simulink library "GOcontroll_Moduline_Target"  (R2023b)
settings: Solver=ode45  StartTime=0.0  StopTime=10.0  RelTol=1e-3  EnableMultiTasking=on
PreLoadFcn:
  | compile_gocontroll_mex;
values from neighbouring files (symbols this model uses):
  id = 2    [sfcn_UDPReceive.m]    (also in sfcn_UDPSend.m = 4)
undefined symbols (not defined in the file or in its folder): C_Cb1Pt10, Cb1Pt10_RAW_ERR_HIGH, Cb1Pt10_RAW_ERR_LOW, Cb1Pt10_SIG_ERR_HIGH, Cb1Pt10_SIG_ERR_LOW, Cb1Pt10_SIG_WAR_HIGH, Cb1Pt10_SIG_WAR_LOW, Pres_0_20_bar_500_4500_mv_inv, signal_x_RAW_ERR_HIGH, signal_x_RAW_ERR_LOW, signal_x_SIG_ERR_HIGH, signal_x_SIG_ERR_LOW, signal_x_SIG_WAR_HIGH, signal_x_SIG_WAR_LOW, signal_x_SPN, Valve1_ACTIVE_DUTY_CYCLE, Valve1_MAX_CURRENT, Valve1_MIN_CURRENT, Valve1_SPN
libraries: $bdroot x17, simulink x12, canmsglib x4
(part 4 of 5)

== system GOcontroll_Moduline_Target/Network/TCP ==
  TCP Configure : M-S-Function  FunctionName=sfcn_TCPConfig  mask(TCP Configure){socket_id=id, port=9001, ip='0.0.0.0', socket_mode=Server, remote_port=9002, remote_ip='0.0.0.0', timeout=1000}
      mask prompts: socket_id "Socket id"; port "The port on which to listen/send"; ip "The ip on which to listen/send"; socket_mode "Socket mode:"; remote_port "The port to connect to"; remote_ip "The ip to connect to"; timeout "The connection timeout (ms)"
      mask help:
      | Block to configure a TCP socket
      |
      | The socket ID should be a unique identifier to link the send and receive blocks to.
      | The name of the actual socket in the C code will be socket_<socket id>, so characters that would not work in a C variable name will not work.
      |
      | Setting the ip to 0.0.0.0 makes the controller accept messages on all interfaces.
      | Set it to the ip of a specific interface to limit this.
      |
      | The socket mode determines whether this socket will listen for a connection or actively try to make one to a given ip and port.
      | Server will wait for something to connect to it, the client will try to connect to a server at the given ip and port
      |
      | Setting the timeout to zero disables the timeout
      |
      | When the disconnect input is true, it will close the current connection if there is one, if there isn't one it will not allow a connection to be made as long as it is true.
      |
      | Outputs whether or not the socket currently has an active connection (true means connnected)
      mask init:
      | if ~is_ip(ip)
      |         error('Entered IP is not valid');
      |     end
      |     if mod(port,1) > 0 || port < intmin('uint16') || port > intmax('uint16')
      |         error('Entered Port is not valid, it should be an integer from 0-65335');
      |     end
      | 
      |     if ~is_ip(remote_ip)
      |         error('Entered remote IP is not valid');
      |     end
      |     if mod(remote_port,1) > 0 || remote_port < intmin('uint16') || remote_port > intmax('uint16')
      |         error('Entered remote Port is not valid, it should be an integer from 0-65335');
      |     end
      | 
      |     if mod(timeout,1) > 0 || timeout < intmin('uint32') || timeout > intmax('uint32')
      |         error('Entered timeout is not valid, it should be an integer from 0-4.294.967.295');
      |     end
      | 
      |     blockPath = split(gcb, '/');
      |     configures = find_system(blockPath(1),'RegExp', 'on','FollowLinks', 'on','MaskType','TCP Configure');
      |     options = cell(1,length(configures));
      |     for idx = 1:length(configures)
      |         options(idx) = get_param(configures(idx),'socket_id');
      |     end
      | 
      |     if length(unique(options)) ~= length(options)
      |         error('Socket id is already in use, set a unique socket id');
      |     end
      | 
      | 	modelRTWFields = struct('port', num2str(port), 'ip', ip, 'socket_id', socket_id, ...
      |         'remote_port', num2str(remote_port), 'remote_ip', remote_ip, 'socket_mode', num2str(socket_mode), 'timeout', num2str(timeout));
      | 
      | 	% Insert modelRTWFields in the I/O block S-Function containing the Tag starting with 'HANcoder_TARGET_'
      | 	HANcoder_TARGET_DataBlock = find_system(gcb, 'RegExp', 'on', 'FollowLinks', 'on', 'LookUnderMasks', 'all', 'BlockType', 'M-S-Function');
      | 	set_param(HANcoder_TARGET_DataBlock{1}, 'RTWdata', modelRTWFields);
      mask TypeOptions socket_mode: Server | Client
      mask Callback socket_mode:
      | mode = get_param(gcb, 'socket_mode');
      | mask = Simulink.Mask.get(gcb);
      | pars = mask.Parameters;
      | if strcmp(mode, 'Server')
      |     pars(5).set('Visible', 'off');
      |     pars(6).set('Visible', 'off');
      | else
      |     pars(5).set('Visible', 'on');
      |     pars(6).set('Visible', 'on');
      | end
      mask Display:
      | if (socket_mode == 1)
      |     fprintf('Configure TCP server\n IP: %s\nPort: %d',ip,port);
      | else
      |     fprintf('Configure TCP client\n IP: %s\nPort: %d\nRemote IP: %s\n Remote port: %d',ip,port,remote_ip,remote_port);
      | end
      | port_label('output', 1, 'connected');
      | port_label('input', 1, 'disconnect');
      | text(2, 6, ert_linux_target_version());
  TCP Receive : S-Function  FunctionName=sfcn_TCPReceive  Parameters=buff_len,socket_mode,socket_id,tsamp  SFunctionDeploymentMode=off  EnableBusSupport=off  mask(TCP Receive){tsamp=-1, socket_id=id, buff_len=1, socket_mode=Server}
      mask prompts: tsamp "Sample time"; socket_id "Socket"; buff_len "Buffer size"
      mask help:
      | Receive all TCP messages on the given socket
      |
      | For every message received this block will call the functions attached to the function call output.
      | In these function calls you can then use the message and message length outputs to process/buffer the received messages.
      |
      | Outputs:
      | function call:
      | Attach to a function call subsystem or something like it to call that function every time a message is received.
      |
      | message:
      | The uint8 vector received from the socket. The length of this vector is likely longer than the actual number of bytes received.
      |
      | message length:
      | The number of bytes actually received, use this to get the actual fresh bytes from the message.
      |
      | Parameters:
      | buffer size:
      | The maximum number of bytes that can be read from the socket in one message, this also determines the width of the message vector.
      mask TypeOptions socket_id: id
      mask Callback socket_id:
      | blockPath = split(gcb, '/');
      | configures = find_system(blockPath(1),'RegExp', 'on','FollowLinks', 'on','MaskType','TCP Configure');
      | mask = Simulink.Mask.get(gcb);
      | pars = mask.Parameters;
      | options = cell(1,length(configures));
      | for idx = 1:length(configures)
      |     options(idx) = get_param(configures(idx),'socket_id');
      | end
      | mask.getParameter('socket_id').TypeOptions = options;
      | for idx = 1:length(configures)
      |     if strcmp(get_param(configures(idx),'socket_id'), get_param(gcb, 'socket_id'))
      |         mode = Simulink.Mask.get(configures{idx}).getParameter('socket_mode').Value;
      |         set_param(gcb, 'socket_mode', mode);
      |     end
      | end
      mask TypeOptions socket_mode: Server | Client
      mask Display:
      | fprintf('TCP Receive\nSocket: %s', socket_id);
      | text(2, 6, ert_linux_target_version());
      | port_label('output', 1, 'function call');
      | port_label('output', 2, 'message');
      | port_label('output', 3, 'message length');
  TCP Send : M-S-Function  FunctionName=sfcn_TCPSend  Parameters=tsamp  mask(TCP Send){socket_id=id, tsamp=1, socket_mode=Server}
      mask prompts: socket_id "Socket"; tsamp "Sample time"
      mask help:
      | Send a TCP message to the chosen sockets connection, whether it be client or server.
      |
      | The Message input should be a uint8 vector, if you end up with a [1xn] or [nx1] matrix, use the reshape block to turn it into a vector.
      mask init:
      | % update RTWdata to call WriteRTW again
      |     modelRTWFields = struct('socket_id', socket_id, 'socket_mode', num2str(socket_mode));
      | 
      |     % Insert modelRTWFields in the I/O block S-Function containing the Tag starting with 'HANcoder_TARGET_'
      |     HANcoder_TARGET_DataBlock = find_system(gcb, 'RegExp', 'on', 'FollowLinks', 'on', 'LookUnderMasks', 'all', 'BlockType', 'M-S-Function');
      |     set_param(HANcoder_TARGET_DataBlock{1}, 'RTWdata', modelRTWFields);
      mask TypeOptions socket_id: id
      mask Callback socket_id:
      | blockPath = split(gcb, '/');
      | configures = find_system(blockPath(1),'RegExp', 'on','FollowLinks', 'on','MaskType','TCP Configure');
      | mask = Simulink.Mask.get(gcb);
      | pars = mask.Parameters;
      | options = cell(1,length(configures));
      | for idx = 1:length(configures)
      |     options(idx) = get_param(configures(idx),'socket_id');
      | end
      | mask.getParameter('socket_id').TypeOptions = options;
      | for idx = 1:length(configures)
      |     if strcmp(get_param(configures(idx),'socket_id'), get_param(gcb, 'socket_id'))
      |         mode = Simulink.Mask.get(configures{idx}).getParameter('socket_mode').Value;
      |         set_param(gcb, 'socket_mode', mode);
      |     end
      | end
      mask TypeOptions socket_mode: Server | Client
      mask Display:
      | fprintf('TCP Send\nSocket: %s',socket_id);
      | port_label('input', 1, 'message');
      | text(2, 6, ert_linux_target_version());

== system GOcontroll_Moduline_Target/Network/UDP ==
  UDP Configure : M-S-Function  FunctionName=sfcn_UDPConfig  mask(UDP Configure){socket_id=id, port=9001, ip='0.0.0.0', broadcast=on}
      mask prompts: socket_id "Socket id"; port "The port on which to listen/send"; ip "The ip on which to listen/send"; broadcast "Allow broadcasting of sent messages"
      mask help:
      | Block to configure a UDP connection
      |
      | The socket ID should be a unique identifier to link the send and receive blocks to.
      | The name of the actual socket in the C code will be socket_<socket id>, so characters that would not work in a C variable name will not work.
      |
      | Setting the ip to 0.0.0.0 makes the controller accept messages on all interfaces.
      | Set it to the ip of a specific interface to limit this.
      |
      | Allowing broadcasting enables you to send messages to a full range of ip addresses, for example:
      | 192.168.255.255 sends messages to 192.168.1.1, 192.168.2.1 ... 192.168.1.2, 192.168.1.3...
      mask init:
      | if broadcast == 0
      |         broadcastStr = "Not broadcasting";
      |     else
      |         broadcastStr = "Broadcasting";
      |     end
      |     if ~is_ip(ip)
      |         error('Entered IP is not valid');
      |     end
      |     if mod(port,1) > 0 || port < intmin('uint16') || port > intmax('uint16')
      |         error('Entered Port is not valid, it should be an integer from 0-65335');
      |     end
      | 
      |     blockPath = split(gcb, '/');
      |     configures = find_system(blockPath(1),'RegExp', 'on','FollowLinks', 'on','MaskType','UDP Configure');
      |     options = cell(1,length(configures));
      |     for idx = 1:length(configures)
      |         options(idx) = get_param(configures(idx),'socket_id');
      |     end
      | 
      |     if length(unique(options)) ~= length(options)
      |         error('Socket id is already in use, set a unique socket id');
      |     end
      | 
      | 	modelRTWFields = struct('port', num2str(port), 'ip', ip, 'broadcast', num2str(broadcast), 'socket_id', socket_id);
      | 
      | 	% Insert modelRTWFields in the I/O block S-Function containing the Tag starting with 'HANcoder_TARGET_'
      | 	HANcoder_TARGET_DataBlock = find_system(gcb, 'RegExp', 'on', 'FollowLinks', 'on', 'LookUnderMasks', 'all', 'BlockType', 'M-S-Function');
      | 	set_param(HANcoder_TARGET_DataBlock{1}, 'RTWdata', modelRTWFields);
      mask Display:
      | fprintf('Configure UDP socket\n IP: %s\nPort: %d\n%s',ip,port,broadcastStr);
      | text(2, 6, ert_linux_target_version());
  UDP Example : Subsystem
  UDP Receive : S-Function  FunctionName=sfcn_UDPReceive  Parameters=buff_len,socket_id,tsamp  SFunctionDeploymentMode=off  EnableBusSupport=off  mask(UDP Receive){tsamp=-1, socket_id=id, buff_len=1}
      mask prompts: tsamp "Sample time"; socket_id "Socket"; buff_len "Buffer size"
      mask help:
      | Receive all UDP messages
      |
      | For every message received this block will call the functions attached to the function call output.
      | In these function calls you can then use the message and message length outputs to process/buffer the received messages.
      |
      | Outputs:
      | function call:
      | Attach to a function call subsystem or something like it to call that function every time a message is received.
      |
      | message:
      | The uint8 vector received from the socket. The length of this vector is likely longer than the actual number of bytes received.
      |
      | message length:
      | The number of bytes actually received, use this to get the actual fresh bytes from the message.
      |
      | Parameters:
      | buffer size:
      | The maximum number of bytes that can be read from the socket in one message, this also determines the width of the message vector.
      mask TypeOptions socket_id: id | led_sinus
      mask Callback socket_id:
      | blockPath = split(gcb, '/');
      | configures = find_system(blockPath(1),'RegExp', 'on','FollowLinks', 'on','MaskType','UDP Configure');
      | mask = Simulink.Mask.get(gcb);
      | pars = mask.Parameters;
      | options = cell(1,length(configures));
      | for idx = 1:length(configures)
      |     options(idx) = get_param(configures(idx),'socket_id');
      | end
      | mask.getParameter('socket_id').TypeOptions = options;
      mask Display:
      | fprintf('UDP Receive');
      | text(2, 6, ert_linux_target_version());
      | port_label('output', 1, 'function call');
      | port_label('output', 2, 'message');
      | port_label('output', 3, 'message length');
  UDP Send : M-S-Function  FunctionName=sfcn_UDPSend  Parameters=tsamp,ip,port  mask(UDP Send){socket_id=id, ip='0.0.0.0', port=9001, tsamp=1}
      mask prompts: socket_id "Socket"; ip "The IP address to send to"; port "The port to send to"; tsamp "Sample time"
      mask help:
      | Send a UDP message to the designated address.
      |
      | The Message input should be a uint8 vector, if you end up with a [1xn] or [nx1] matrix, use the reshape block to turn it into a vector.
      |
      | IP address should be a valid IP address as a string
      |
      | Port should be a within the range of a uint16
      mask init:
      | if ~is_ip(ip)
      |         error('Entered IP is not valid');
      |     end
      |     if mod(port,1) > 0 || port < intmin('uint16') || port > intmax('uint16')
      |         error('Entered Port is not valid, it should be an integer from 0-65335');
      |     end
      |     % update RTWdata to call WriteRTW again
      |     modelRTWFields = struct('port', num2str(port), 'ip', ip, 'socket_id', socket_id);
      | 
      |     % Insert modelRTWFields in the I/O block S-Function containing the Tag starting with 'HANcoder_TARGET_'
      |     HANcoder_TARGET_DataBlock = find_system(gcb, 'RegExp', 'on', 'FollowLinks', 'on', 'LookUnderMasks', 'all', 'BlockType', 'M-S-Function');
      |     set_param(HANcoder_TARGET_DataBlock{1}, 'RTWdata', modelRTWFields);
      mask TypeOptions socket_id: id | led_sinus
      mask Callback socket_id:
      | blockPath = split(gcb, '/');
      | configures = find_system(blockPath(1),'RegExp', 'on','FollowLinks', 'on','MaskType','UDP Configure');
      | mask = Simulink.Mask.get(gcb);
      | pars = mask.Parameters;
      | options = cell(1,length(configures));
      | for idx = 1:length(configures)
      |     options(idx) = get_param(configures(idx),'socket_id');
      | end
      | pars(1).TypeOptions = options;
      mask Display:
      | fprintf('UDP Send\nIP: %s\nPort: %d',ip,port);
      | port_label('input', 1, 'message');
      | text(2, 6, ert_linux_target_version());

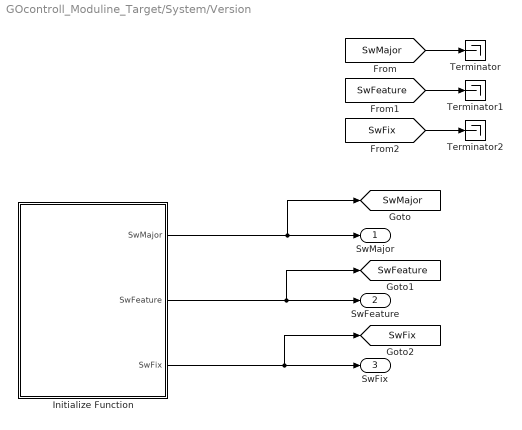
== system GOcontroll_Moduline_Target/System/Version ==
  Initialize Function : Subsystem  TreatAsAtomicUnit=on
  Terminator : Terminator
  Terminator1 : Terminator
  Terminator2 : Terminator
  SwMajor : Outport
  SwFeature : Outport  Port=2
  SwFix : Outport  Port=3
  tag scope: SwFeature=global, SwFix=global, SwMajor=global
  wires:
  Initialize Function/2(SwFeature) -> [SwFeature], SwFeature/1
  Initialize Function/1(SwMajor) -> SwMajor/1, [SwMajor]
  Initialize Function/3(SwFix) -> [SwFix], SwFix/1
  [SwMajor] -> Terminator/1
  [SwFeature] -> Terminator1/1
  [SwFix] -> Terminator2/1

== system GOcontroll_Moduline_Target/CAN/ CAN Example/Process messages on CAN2 ==
  note: only control the leds when a message has come in, so use enabled subystems
  note: place all your unpack blocks here attached to the CAN_MESSAGE line
  note: status outputs whether a message has been received the last time the block was activated
  In1 : Inport
  function : TriggerPort  TriggerType=function-call  VariantControl=(inherit)  OutputDataType=int8
  CAN Unpack : canmsglib/CAN Unpack  MsgList=(none)  MsgName=CAN Msg  MsgIDType=Standard (11-bit identifier)  MsgIdentifier=10  MsgLength=2  SignalInfo={ 'led1', '0', '8', 'LE', 'unsigned', 'Standard', '0', '1', '0', '-Inf', 'Inf'; 'led2', '8', '8', 'LE', 'unsigned', 'Standard', '0', '1', '0', '-Inf', 'Inf' }  IDPort=off  TimestampPort=off  ErrorPort=off  RemotePort=off  LengthPort=off  StatusPort=on  ApplyMinMax=off
      settings: LibrarySourceBlock=embeddedtargetslib/Host Communication/CAN Unpack
  CAN Unpack1 : canmsglib/CAN Unpack  MsgList=(none)  MsgName=CAN Msg  MsgIDType=Standard (11-bit identifier)  MsgIdentifier=11  MsgLength=2  SignalInfo={ 'led3', '0', '8', 'LE', 'unsigned', 'Standard', '0', '1', '0', '-Inf', 'Inf'; 'led4', '8', '8', 'LE', 'unsigned', 'Standard', '0', '1', '0', '-Inf', 'Inf' }  IDPort=off  TimestampPort=off  ErrorPort=off  RemotePort=off  LengthPort=off  StatusPort=on  ApplyMinMax=off
      settings: LibrarySourceBlock=embeddedtargetslib/Host Communication/CAN Unpack
  Control Leds : Subsystem  TreatAsAtomicUnit=on
  Enabled Subsystem : Subsystem  TreatAsAtomicUnit=on
  wires:
  CAN Unpack1/1 -> Enabled Subsystem/1(In4)
  CAN Unpack1/2 -> Enabled Subsystem/2(In2)
  CAN Unpack1/3 -> Enabled Subsystem/Enable
  CAN Unpack/3 -> Control Leds/Enable
  CAN Unpack/1 -> Control Leds/1(In1)
  CAN Unpack/2 -> Control Leds/2(In3)
  In1/1 -> CAN Unpack/1, CAN Unpack1/1

== system GOcontroll_Moduline_Target/Memory store/Diagnostic to memory/Delete all codes for one group ==
  Trigger : TriggerPort  VariantControl=(inherit)  PortDimensions=1
  Delete all DTC from memory : M-S-Function  FunctionName=sfcn_memory_diagnostic_delete_code  mask(Delete diagnostic codes from memory){}
      mask help:
      | This function block deletes all stored codes.
      |
      | Sample time:
      | -1 for inherited since this block is a triggered system
      mask init:
      | % Insert modelRTWFields in the I/O block S-Function containing the Tag starting with 'HANcoder_TARGET_'
      | HANcoder_TARGET_DataBlock = find_system(gcb, 'RegExp', 'on', 'FollowLinks', 'on', 'LookUnderMasks', 'all', 'BlockType', 'M-S-Function');
      mask Display:
      | fprintf('Delete all DTCs from memory');
      | text(2, 6, ert_linux_target_version());

== system GOcontroll_Moduline_Target/Memory store/Diagnostic to memory/Delete single DTC code ==
  In1 : Inport
  In2 : Inport  Port=2
  Trigger : TriggerPort  VariantControl=(inherit)
  Delete diagnostic code : M-S-Function  FunctionName=sfcn_memory_diagnostic_delete_single_code  mask(Store diagnostic code to memory){}
      mask help:
      | This function block stores a diagnostic code to memory.
      |
      | Diagnostic code type:
      | The type defines the severity of the diagnostic code.
      |
      | This block should be placed in a triggered subsystem
      mask init:
      | % Insert modelRTWFields in the I/O block S-Function containing the Tag starting with 'HANcoder_TARGET_'
      | HANcoder_TARGET_DataBlock = find_system(gcb, 'RegExp', 'on', 'FollowLinks', 'on', 'LookUnderMasks', 'all', 'BlockType', 'M-S-Function');
      mask Display:
      | fprintf('Delete single DTC from memory');
      | port_label('input', 1, 'SPN');
      | port_label('input', 2, 'FMI');
      | text(2, 6, ert_linux_target_version());
  wires:
  In2/1 -> Delete diagnostic code/2
  In1/1 -> Delete diagnostic code/1

== system GOcontroll_Moduline_Target/Memory store/Diagnostic to memory/Diagnostic Helpers ==
  Actuator diagnostic : Subsystem  mask(Generic actuator diagnostic block){delay=1000, duration=2000, actuatorName=Valve1, spn=Valve1_SPN}
      mask prompts: delay "Start delay [ms]"; duration "Fault duration [ms]"; actuatorName "Actuator name:"
      mask help:
      | This block executes diagnostics on an actuator that goes into the block. The current during control is checked.
      |
      | It must be enabled via the enable input at the top to function, this can be a easy way to toggle diagnostics on or off.
      |
      | To use this block, error limits should be defined in the workspace. Several pre- and suffixes are needed to work with this block. For example:
      |
      | Base actuator name is: Valve1 (this will be the signal name in the mask)
      |
      | - Valve1_ACTIVE_DUTY_CYCLE (This is the dutycycle when the valve is controlles. in case a switch is used, use 1)
      | - Valve1_MIN_CURRENT (Current in mA that should be the minimal to control the valve)
      | - Valve1_MAX_CURRENT (Current in mA that should be the minimal to control the valve)
      |
      | Setting Diagnostic Trouble Code (DTC) in memory:
      |
      | Configure the SPN number corresponding to the signal in the workspace parameters as:
      | Valve1_SPN
      |
      | Output provide two uint8 signals in a bus holding the volatile and permanent fault flags.
      mask Callback actuatorName:
      | set_param(gcb, 'MaskSelfModifiable', 'on');
      | 
      | S = get_param(gcb,"actuatorName");
      | set_param(gcb + "/ActiveState",'const', S + "_ACTIVE_DUTY_CYCLE");
      | set_param(gcb + "/ActiveState2",'const', S + "_ACTIVE_DUTY_CYCLE");
      | set_param(gcb + "/MinimalCurrent",'const', S + "_MIN_CURRENT");
      | set_param(gcb + "/MaximalCurrent",'const', S + "_MAX_CURRENT");
      | 
      | set_param(gcb, 'spn', S + "_SPN");
      | 
      | % Set signal naming
      | P = get_param(gcb + "/Per",'PortHandles');
      | PerSubOut = P.Outport(1);
      | l1 = get_param(PerSubOut,'Line');
      | set_param(l1,'Name',"Per_" + S);
      | 
      | V = get_param(gcb + "/Vol",'PortHandles');
      | VolSubOut = V.Outport(1);
      | l1 = get_param(VolSubOut,'Line');
      | set_param(l1,'Name',"Vol_" + S);
      | 
      | try
      |     O = get_param(gcb,'PortHandles');
      |     PortOut = O.Outport(1);
      |     l1 = get_param(PortOut,'Line');
      |     set_param(l1,'Name',S);
      | end
      mask DialogControl ParameterGroupVar Prompt: Diagnostic parameters
      mask Display:
      | fprintf('%s\n SPN: %d',...
      |     actuatorName,spn);
      | 
      | port_label('input', 1, 'Reset');
      | port_label('input', 2, 'Duty cycle [0-1000]');
      | port_label('input', 3, 'Measured current [mA]');
      | 
      | text(2, 6, ert_linux_target_version());
  Diagnostic simulation : Subsystem  mask(Diagnostic simulation){signalName=Cb1Pt10, sensorCurveText=Pres_0_20_bar_500_4500_mv_inv, sensorCurve=Pres_0_20_bar_500_4500_mv_inv}
      mask prompts: signalName "Signal"; sensorCurveText "Sensor curve"
      mask help:
      | This block works together with the "Signal adaptation" and "Signal diagnostic" blocks to provide an easy way to test the setting of diagnostic codes for analogue inputs.
      |
      | It needs both of those blocks to be properly set up in the model along with their workspace variables. Then the Simulation variable of this signal must be set to 1.
      |
      | A diagnostic scenario can then be injected:
      | == 1/default: normal operation
      | == 2: low voltage
      | == 3: high voltage
      | == 4: too low error
      | == 5: too high error
      | == 6: too low warning
      | == 7: too high warning
      |
      | To simulate this it requires an extra lookup table which is the inverse of the normal signal lookup table, it should transfor the real world value back into the raw input.
      mask Callback signalName:
      | set_param(gcb, 'MaskSelfModifiable', 'on');
      | 
      | S = get_param(gcb,"signalName");
      |  set_param(gcb + "/LowVoltage", 'Value', S + "_RAW_ERR_LOW -1");
      |  set_param(gcb + "/HighVoltage", 'Value', S + "_RAW_ERR_HIGH +1");
      |  set_param(gcb + "/LowWarning",  'Value',S + "_SIG_WAR_LOW -1");
      |  set_param(gcb + "/HighWarning", 'Value', S + "_SIG_WAR_HIGH +1");
      |  set_param(gcb + "/LowError", 'Value', S + "_SIG_ERR_LOW -1");
      |  set_param(gcb + "/HighError", 'Value', S + "_SIG_ERR_HIGH +1");
      |  set_param(gcb + "/Normal", 'Value', "C_" + S);
      | 
      | % Set Goto tags depending on signal naming
      | set_param(gcb + "/ToRaw","GotoTag","RawSim_" + S);
      | set_param(gcb, "sensorCurve", get_param(gcb,"sensorCurveText"));
      mask Display:
      | fprintf('%s', signalName);
      | 
      | text(2, 6, ert_linux_target_version());
  Generic diagnostic : Subsystem  mask(Generic actuator diagnostic block){delay=1000, duration=2000, naming=Valve2, spn=1234, fmi=(0) Data valid but above normal operational range, most severe level (3)}
      mask prompts: delay "Start delay [ms]"; duration "Fault duration [ms]"; spn "SPN number"; fmi "Failure Mode Indicator"
      mask help:
      | A simple diagnostic helper, diagnostics start after "Start delay" and then if trigger == 1 for "Fault duration" it will write the fault code to memory.
      |
      | Once the trigger drops to 0 again, the volatile output will also go back to 0, but the persistant output will remain at 1. Untill the reset input is applied, this will also reset the persistant output. Note that this will not delete the code from memory.
      |
      | The naming parameter is non functional but helps by naming the output signals and being displayed in the mask.
      mask Callback naming:
      | set_param(gcb, 'MaskSelfModifiable', 'on');
      | 
      | S = get_param(gcb,"naming");
      | 
      | % Set signal naming
      | try
      |     P = get_param(gcb,'PortHandles');
      |     OutputPort1 = P.Outport(1);
      |     l1 = get_param(OutputPort1,'Line');
      |     set_param(l1,'Name',"Per_" + S);
      | 
      |     OutputPort2 = P.Outport(2);
      |     l1 = get_param(OutputPort2,'Line');
      |     set_param(l1,'Name',"Vol_" + S);
      | end
      mask TypeOptions spn: Store diagnostic code/spn
      mask TypeOptions fmi: Store diagnostic code/fmi
      mask DialogControl ParameterGroupVar Prompt: Diagnostic parameters
      mask Display:
      | fprintf('%s\n\nDTC serverity: %d\nSPN: %d',...
      |     naming,fmi,spn);
      | 
      | port_label('input', 1, 'Reset');
      | port_label('input', 2, 'Trigger');
      | 
      | port_label('output', 1, 'Persistant flag');
      | port_label('output', 2, 'Volatile flag');
      | 
      | text(2, 6, ert_linux_target_version());
  Signal diagnostic : Subsystem  mask(Generic Signal diagnostic block){delay=1000, duration=1000, signalName=signal_x, spn=signal_x_SPN}
      mask prompts: delay "Start delay [ms]"; duration "Fault duration [ms]"; signalName "Signal name:"
      mask help:
      | This block executes diagnostics on a signal that goes into the block. Both sensor voltage and signal thersholds are checked.
      |
      | It must be enabled via the enable input at the top to function, this can be a easy way to toggle diagnostics on or off.
      |
      | To use this block, error and warning limits should be defined in the workspace. Several pre- and suffixes are needed to work with this block. For example:
      |
      | Base signal name is: Coolant_Pt1 (this will be the signal name in the mask)
      |
      | - Coolant_Pt1_RAW_ERR_LOW (low voltage error)
      | - Coolant_Pt1_RAW_ERR_HIGH (high voltage error)
      | - Coolant_Pt1_SIG_WAR_LOW (Low warning signal threshold)
      | - Coolant_Pt1_SIG_WAR_HIGH (High warning signal threshold)
      | - Coolant_Pt1_SIG_ERR_LOW (Low error signal threshold)
      | - Coolant_Pt1 _SIG_ERR_HIGH (High error signal threshold)
      |
      | Setting Diagnostic Trouble Code (DTC) in memory:
      |
      | Configure the SPN number corresponding to the signal in the workspace parameters as:
      | Coolant_Pt1_SPN
      |
      | Output provide two uint8 signals in a bus holding the volatile and permanent fault flags.
      mask Callback signalName:
      | set_param(gcb, 'MaskSelfModifiable', 'on');
      | 
      | S = get_param(gcb,"signalName");
      | set_param(gcb + "/LowVoltage",'const', S + "_RAW_ERR_LOW");
      | set_param(gcb + "/HighVoltage",'const', S + "_RAW_ERR_HIGH");
      | set_param(gcb + "/LowWarning",'const', S + "_SIG_WAR_LOW");
      | set_param(gcb + "/HighWarning",'const', S + "_SIG_WAR_HIGH");
      | set_param(gcb + "/LowError",'const', S + "_SIG_ERR_LOW");
      | set_param(gcb + "/HighError",'const', S + "_SIG_ERR_HIGH");
      | 
      | set_param(gcb,'spn', S + "_SPN");
      | 
      | % Set signal naming
      | P = get_param(gcb + "/Per",'PortHandles');
      | PerSubOut = P.Outport(1);
      | l1 = get_param(PerSubOut,'Line');
      | set_param(l1,'Name',"Per_" + S);
      | 
      | V = get_param(gcb + "/Vol",'PortHandles');
      | VolSubOut = V.Outport(1);
      | l1 = get_param(VolSubOut,'Line');
      | set_param(l1,'Name',"Vol_" + S);
      | 
      | try
      |     O = get_param(gcb,'PortHandles');
      |     PortOut = O.Outport(1);
      |     l1 = get_param(PortOut,'Line');
      |     set_param(l1,'Name',S);
      | end
      mask DialogControl ParameterGroupVar Prompt: Diagnostic parameters
      mask Display:
      | fprintf('%s\nSPN: %d',...
      |     signalName,spn);
      | 
      | port_label('input', 1, 'Reset');
      | port_label('input', 2, 'RAW signal');
      | port_label('input', 3, 'Physical signal');
      | 
      | text(2, 6, ert_linux_target_version());

== system GOcontroll_Moduline_Target/Memory store/Diagnostic to memory/Store diagnostic code ==
  Trigger : TriggerPort  VariantControl=(inherit)
  Store DTC code : M-S-Function  FunctionName=sfcn_memory_diagnostic_write_code  mask(Store diagnostic code to memory){spn=spn, fmi=(0) Data valid but above normal operational range, most severe level (3)}
      mask prompts: spn "SPN number"; fmi "Failure Mode Indicator"
      mask help:
      | This function block stores a diagnostic code to memory.
      |
      | SPN number:
      | A code to identify which part has failed
      |
      | FMI:
      | How the part has failed
      |
      | This block should be placed in a triggered subsystem
      mask init:
      | % Create resource keywords to be reserved in resource database
      | modelRTWFields = 	struct(	'spn',int2str(spn),'fmi',int2str(fmi));
      | 
      | % Insert modelRTWFields in the I/O block S-Function containing the Tag starting with 'HANcoder_TARGET_'
      | HANcoder_TARGET_DataBlock = find_system(gcb, 'RegExp', 'on', 'FollowLinks', 'on', 'LookUnderMasks', 'all', 'BlockType', 'M-S-Function');
      | set_param(HANcoder_TARGET_DataBlock{1}, 'RTWdata', modelRTWFields);
      mask Display:
      | fprintf('Store DTC in memory\n SPN: %s\nFMI: %s',spn,fmi);
      | text(2, 6, ert_linux_target_version());

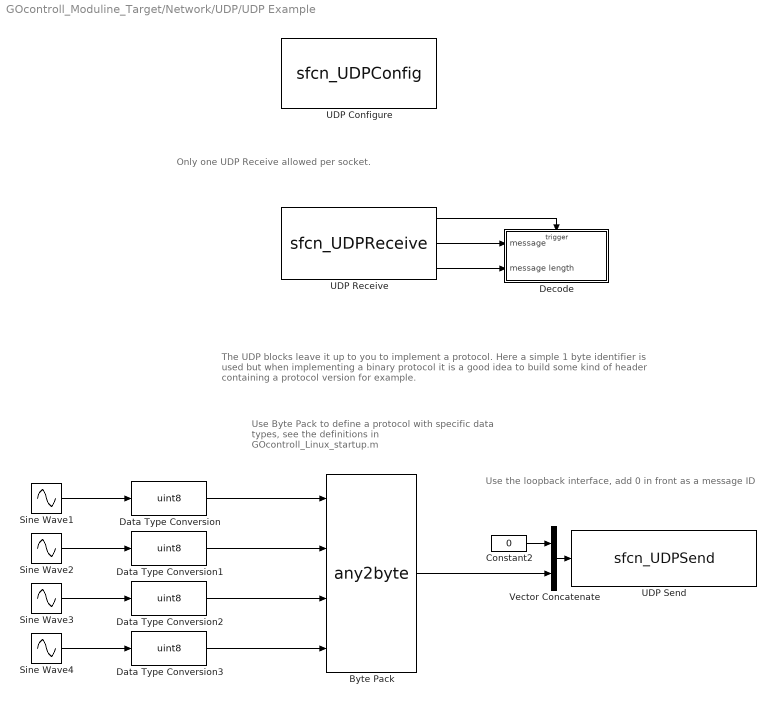
== system GOcontroll_Moduline_Target/Network/UDP/UDP Example ==
  note: The UDP blocks leave it up to you to implement a protocol.
      | Here a simple 1 byte identifier is used but when implementing a binary protocol
      | it is a good idea to build some kind of header containing a protocol version for example.
  note: Only one UDP Receive allowed per socket.
  note: Use Byte Pack to define a protocol with
      | specific data types, see the definitions in
      | GOcontroll_Linux_startup.m
  note: Use the loopback interface, add 0 in front as  a
      | message ID
  Byte Pack : S-Function  AncestorBlock=etargetslib/Byte Pack  FunctionName=any2byte  Parameters=datatypesout,byteAlign  SFunctionDeploymentMode=off  EnableBusSupport=off  mask(Byte pack){datatypes={'uint8','uint8','uint8','uint8'}, byteAlign=1}
      mask prompts: datatypes "Input port data types (cell array):"; byteAlign "Byte alignment:"
      mask help: Pack input data into a single output vector of type uint8. Insert before a UDP Send block to produce a uint8 byte vector from multiple vectors of varying data type.
      mask init:
      | datatypesout = bytepack_callback(datatypes);
      mask Help: eval('linkfoundation.util.openBlockHelp(''etargetslibbytepack'')');
      mask TypeOptions byteAlign: 1 | 2 | 4 | 8
      mask Display:
      | color('blue');
      | text(0.95, 0.90, '', ...
      |                 'horizontalalignment', 'right');
      | color('black');
      | text(0.50, 0.12, 'Byte Pack', ...
      |                 'horizontalAlignment','center');
  Constant2 : Constant  Value=0  OutDataTypeStr=uint8
  Data Type Conversion{,1..3} (4 alike) : DataTypeConversion  OutDataTypeStr=uint8  SaturateOnIntegerOverflow=off  RndMeth=Floor
  Decode : Subsystem  TreatAsAtomicUnit=on
  Sine Wave{1..4} (4 alike) : Sin  SineType=Sample based  Amplitude=120  Bias=121  Phase=128  Samples=100  SampleTime=0.01
  UDP Configure : M-S-Function  AncestorBlock=GOcontroll_Moduline_Target/Network/UDP/UDP Configure  FunctionName=sfcn_UDPConfig  mask(UDP Configure){socket_id=led_sinus, port=9001, ip='0.0.0.0', broadcast=off}
      mask prompts: socket_id "Socket id"; port "The port on which to listen/send"; ip "The ip on which to listen/send"; broadcast "Allow broadcasting of sent messages"
      mask help:
      | Block to configure a UDP connection
      |
      | Setting the ip to 0.0.0.0 makes the controller accept messages on all interfaces.
      | Set it to the ip of a specific interface to limit this.
      |
      | Allowing broadcasting enables you to send messages to a full range of ip addresses, for example:
      | 192.168.255.255 sends messages to 192.168.1.1, 192.168.2.1 ... 192.168.1.2, 192.168.1.3...
      mask init: same as GOcontroll_Moduline_Target/Network/UDP/UDP Configure
      mask Display:
      | fprintf('Configure UDP socket\n IP: %s\nPort: %d\n%s',ip,port,broadcastStr);
      | text(2, 6, ert_linux_target_version());
  UDP Receive : S-Function  AncestorBlock=GOcontroll_Moduline_Target/Network/UDP/UDP Receive  FunctionName=sfcn_UDPReceive  Parameters=buff_len,socket_id,tsamp  SFunctionDeploymentMode=off  EnableBusSupport=off  mask(UDP Receive){tsamp=-1, socket_id=led_sinus, buff_len=5}
      mask prompts: tsamp "Sample time"; socket_id "Socket"; buff_len "Buffer size"
      mask help:
      | Receive all UDP messages
      |
      | For every message received this block will call the functions attached to the function call output.
      | In these function calls you can then use the message and message length outputs to process/buffer the received messages.
      |
      | Outputs:
      | function call:
      | Attach to a function call subsystem or something like it to call that function every time a message is received.
      |
      | message:
      | The uint8 vector received from the socket. The length of this vector is likely longer than the actual number of bytes received.
      |
      | message length:
      | The number of bytes actually received, use this to get the actual fresh bytes from the message.
      |
      | Parameters:
      | buffer size:
      | The maximum number of bytes that can be read from the socket in one message, this also determines the width of the message vector.
      mask TypeOptions socket_id: id | led_sinus
      mask Callback socket_id:
      | blockPath = split(gcb, '/');
      | configures = find_system(blockPath(1),'RegExp', 'on','FollowLinks', 'on','MaskType','UDP Configure');
      | mask = Simulink.Mask.get(gcb);
      | pars = mask.Parameters;
      | options = cell(1,length(configures));
      | for idx = 1:length(configures)
      |     options(idx) = get_param(configures(idx),'socket_id');
      | end
      | mask.getParameter('socket_id').TypeOptions = options;
      mask Display:
      | fprintf('UDP Receive');
      | text(2, 6, ert_linux_target_version());
      | port_label('output', 1, 'function call');
      | port_label('output', 2, 'message');
      | port_label('output', 3, 'message length');
  UDP Send : M-S-Function  AncestorBlock=GOcontroll_Moduline_Target/Network/UDP/UDP Send  FunctionName=sfcn_UDPSend  Parameters=tsamp,ip,port  mask(UDP Send){socket_id=led_sinus, ip='127.0.0.1', port=9001, tsamp=0.01}
      mask prompts: socket_id "Socket"; ip "The IP address to send to"; port "The port to send to"; tsamp "Sample time"
      mask help:
      | Send a UDP message to the designated address.
      |
      | The Message input should be a uint8 vector, if you end up with a [1xn] or [nx1] matrix, use the reshape block to turn it into a vector.
      |
      | IP address should be a valid IP address as a string
      |
      | Port should be a within the range of a uint16
      mask init: same as GOcontroll_Moduline_Target/Network/UDP/UDP Send
      mask TypeOptions socket_id: led_sinus
      mask Callback socket_id:
      | blockPath = split(gcb, '/');
      | configures = find_system(blockPath(1),'RegExp', 'on','FollowLinks', 'on','MaskType','UDP Configure');
      | mask = Simulink.Mask.get(gcb);
      | pars = mask.Parameters;
      | options = cell(1,length(configures));
      | for idx = 1:length(configures)
      |     options(idx) = get_param(configures(idx),'socket_id');
      | end
      | pars(1).TypeOptions = options;
      mask Display:
      | fprintf('UDP Send\nIP: %s\nPort: %d',ip,port);
      | port_label('input', 1, 'message');
      | text(2, 6, ert_linux_target_version());
  Vector Concatenate : Concatenate
  wires:
  Vector Concatenate/1 -> UDP Send/1
  UDP Receive/3 -> Decode/2(message length)
  UDP Receive/2 -> Decode/1(message)
  UDP Receive/1 -> Decode/Trigger
  Sine Wave4/1 -> Data Type Conversion3/1
  Sine Wave1/1 -> Data Type Conversion/1
  Constant2/1 -> Vector Concatenate/1
  Sine Wave2/1 -> Data Type Conversion1/1
  Data Type Conversion1/1 -> Byte Pack/2
  Byte Pack/1 -> Vector Concatenate/2
  Data Type Conversion3/1 -> Byte Pack/4
  Sine Wave3/1 -> Data Type Conversion2/1
  Data Type Conversion/1 -> Byte Pack/1
  Data Type Conversion2/1 -> Byte Pack/3

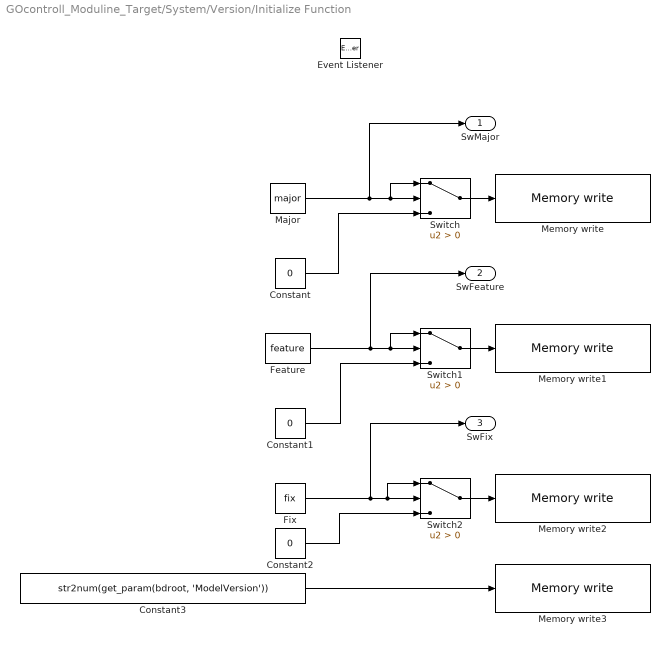
== system GOcontroll_Moduline_Target/System/Version/Initialize Function ==
  Constant : Constant  Value=0  OutDataTypeStr=single
  Constant1 : Constant  Value=0  OutDataTypeStr=single
  Constant2 : Constant  Value=0  OutDataTypeStr=single
  Constant3 : Constant  Value=str2num(get_param(bdroot, 'ModelVersion'))  OutDataTypeStr=single
  Event Listener : EventListener  DisableCoverage=on  EventName=reset
  Feature : Constant  Value=feature  OutDataTypeStr=single
  Fix : Constant  Value=fix  OutDataTypeStr=single
  Major : Constant  Value=major  OutDataTypeStr=single
  Memory write : $bdroot/Memory store/Variable to memory/Memory write  memType=Persistant Memory (eMMC)  tsamp=-1  key=MODEL_MAJOR
  Memory write1 : $bdroot/Memory store/Variable to memory/Memory write  memType=Persistant Memory (eMMC)  tsamp=-1  key=MODEL_FEATURE
  Memory write2 : $bdroot/Memory store/Variable to memory/Memory write  memType=Persistant Memory (eMMC)  tsamp=-1  key=MODEL_FIX
  Memory write3 : $bdroot/Memory store/Variable to memory/Memory write  memType=Persistant Memory (eMMC)  tsamp=-1  key=MODEL_BUILD
  Switch : Switch  Criteria=u2 > Threshold  SaturateOnIntegerOverflow=off  InputSameDT=off
  Switch1 : Switch  Criteria=u2 > Threshold  SaturateOnIntegerOverflow=off  InputSameDT=off
  Switch2 : Switch  Criteria=u2 > Threshold  SaturateOnIntegerOverflow=off  InputSameDT=off
  SwMajor : Outport
  SwFeature : Outport  Port=2
  SwFix : Outport  Port=3
  wires:
  Feature/1 -> Switch1/1, Switch1/2, SwFeature/1
  Constant3/1 -> Memory write3/1
  Fix/1 -> Switch2/1, Switch2/2, SwFix/1
  Major/1 -> Switch/1, Switch/2, SwMajor/1
  Switch/1 -> Memory write/1
  Constant/1 -> Switch/3
  Switch1/1 -> Memory write1/1
  Constant1/1 -> Switch1/3
  Switch2/1 -> Memory write2/1
  Constant2/1 -> Switch2/3

== system GOcontroll_Moduline_Target/CAN/ CAN Example/Process messages on CAN2/Control Leds ==
  In1 : Inport
  In3 : Inport  Port=2
  Enable : EnablePort
  Enclosure LED : $bdroot/Enclosure LED's/Enclosure LED  tsamp=-1  led=1  color=Blue
  Enclosure LED1 : $bdroot/Enclosure LED's/Enclosure LED  tsamp=-1  led=2  color=Blue
  wires:
  In1/1 -> Enclosure LED/1
  In3/1 -> Enclosure LED1/1

== system GOcontroll_Moduline_Target/CAN/ CAN Example/Process messages on CAN2/Enabled Subsystem ==
  In4 : Inport
  In2 : Inport  Port=2
  Enable : EnablePort
  Enclosure LED2 : $bdroot/Enclosure LED's/Enclosure LED  tsamp=-1  led=3  color=Blue
  Enclosure LED3 : $bdroot/Enclosure LED's/Enclosure LED  tsamp=-1  led=4  color=Blue
  wires:
  In4/1 -> Enclosure LED2/1
  In2/1 -> Enclosure LED3/1

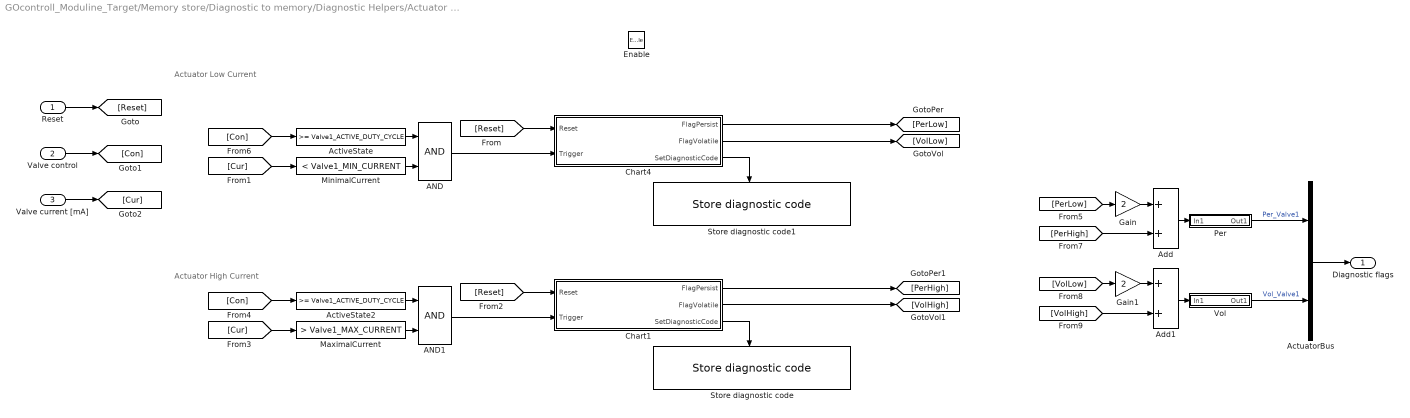
== system GOcontroll_Moduline_Target/Memory store/Diagnostic to memory/Diagnostic Helpers/Actuator diagnostic ==
  note: Actuator Low Current
  note: Actuator High Current
  Reset : Inport
  "Valve control " : Inport  Port=2
  Valve current [mA] : Inport  Port=3
  Enable : EnablePort
  AND : Logic  AllPortsSameDT=off  OutDataTypeStr=boolean
  AND1 : Logic  AllPortsSameDT=off  OutDataTypeStr=boolean
  ActiveState : simulink/Logic and Bit Operations/Compare To Constant  relop=>=  const=Valve1_ACTIVE_DUTY_CYCLE  OutDataTypeStr=boolean
  ActiveState2 : simulink/Logic and Bit Operations/Compare To Constant  relop=>=  const=Valve1_ACTIVE_DUTY_CYCLE  OutDataTypeStr=boolean
  ActuatorBus : BusCreator  Inputs=2
  Add : Sum  OutDataTypeStr=uint8
  Add1 : Sum  AccumDataTypeStr=uint8
  Chart1 : Stateflow chart  TreatAsAtomicUnit=on
  Chart4 : Stateflow chart  TreatAsAtomicUnit=on
  Gain : Gain  Gain=2  OutDataTypeStr=uint8
  Gain1 : Gain  Gain=2  OutDataTypeStr=uint8
  MaximalCurrent : simulink/Logic and Bit Operations/Compare To Constant  relop=>  const=Valve1_MAX_CURRENT  OutDataTypeStr=boolean
  MinimalCurrent : simulink/Logic and Bit Operations/Compare To Constant  relop=<  const=Valve1_MIN_CURRENT  OutDataTypeStr=boolean
  Per : Subsystem
  Store diagnostic code : $bdroot/Memory store/Diagnostic to memory/Store diagnostic code  spn=spn  fmi=(6) Current above normal, or grounded circuit  TriggerType=rising
  Store diagnostic code1 : $bdroot/Memory store/Diagnostic to memory/Store diagnostic code  spn=spn  fmi=(5) Current below normal, or open circuit  TriggerType=rising
  Vol : Subsystem
  Diagnostic flags : Outport  OutputWhenDisabled=reset  InitialOutput=[0]
  wires:
  ActiveState/1 -> AND/1
  MinimalCurrent/1 -> AND/2
  [Cur] -> MinimalCurrent/1
  [Con] -> ActiveState/1
  Chart4/3(SetDiagnosticCode) -> Store diagnostic code1/Trigger
  AND/1 -> Chart4/2(Trigger)
  Reset/1 -> [Reset]
  [Reset] -> Chart4/1(Reset)
  "Valve control "/1 -> [Con]
  Valve current [mA]/1 -> [Cur]
  ActuatorBus/1 -> Diagnostic flags/1
  MaximalCurrent/1 -> AND1/2
  Chart1/2(FlagVolatile) -> [VolHigh]
  [Con] -> ActiveState2/1
  Chart1/1(FlagPersist) -> [PerHigh]
  [Reset] -> Chart1/1(Reset)
  AND1/1 -> Chart1/2(Trigger)
  Chart1/3(SetDiagnosticCode) -> Store diagnostic code/Trigger
  ActiveState2/1 -> AND1/1
  [Cur] -> MaximalCurrent/1
  Add/1 -> Per/1(In1)
  Per/1(Out1) -> ActuatorBus/1  "Per_Valve1"
  Vol/1(Out1) -> ActuatorBus/2  "Vol_Valve1"
  Add1/1 -> Vol/1(In1)
  Chart4/1(FlagPersist) -> [PerLow]
  Chart4/2(FlagVolatile) -> [VolLow]
  [PerLow] -> Gain/1
  Gain/1 -> Add/1
  [VolLow] -> Gain1/1
  Gain1/1 -> Add1/1
  [VolHigh] -> Add1/2
  [PerHigh] -> Add/2

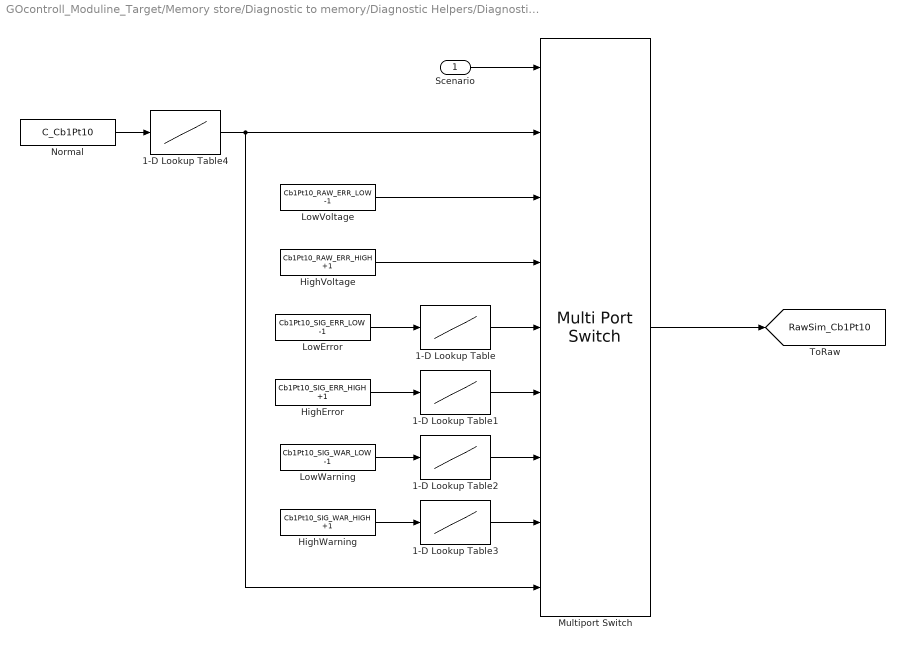
== system GOcontroll_Moduline_Target/Memory store/Diagnostic to memory/Diagnostic Helpers/Diagnostic simulation ==
  Scenario : Inport
  1-D Lookup Table{,1..4} (5 alike) : Lookup_n-D  NumberOfTableDimensions=1  DataSpecification=Lookup table object  LookupTableObject=sensorCurve  BreakpointsForDimension1=[-5:5]  Table=tanh([-5:5])  ExtrapMethod=Clip  InternalRulePriority=Speed  RndMeth=Simplest
  HighError : Constant  Value=Cb1Pt10_SIG_ERR_HIGH +1
  HighVoltage : Constant  Value=Cb1Pt10_RAW_ERR_HIGH +1  OutDataTypeStr=uint16
  HighWarning : Constant  Value=Cb1Pt10_SIG_WAR_HIGH +1
  LowError : Constant  Value=Cb1Pt10_SIG_ERR_LOW -1
  LowVoltage : Constant  Value=Cb1Pt10_RAW_ERR_LOW -1  VectorParams1D=off  OutDataTypeStr=int16
  LowWarning : Constant  Value=Cb1Pt10_SIG_WAR_LOW -1  OutDataTypeStr=single
  Multiport Switch : MultiPortSwitch  Inputs=7  DataPortForDefault=Additional data port  SaturateOnIntegerOverflow=off  InputSameDT=off
  Normal : Constant  Value=C_Cb1Pt10  VectorParams1D=off
  tag scope: RawSim_Cb1Pt10=global
  wires:
  Normal/1 -> 1-D Lookup Table4/1
  1-D Lookup Table4/1 -> Multiport Switch/2, Multiport Switch/9
  1-D Lookup Table1/1 -> Multiport Switch/6
  LowVoltage/1 -> Multiport Switch/3
  Multiport Switch/1 -> [RawSim_Cb1Pt10]
  Scenario/1 -> Multiport Switch/1
  HighVoltage/1 -> Multiport Switch/4
  1-D Lookup Table2/1 -> Multiport Switch/7
  1-D Lookup Table3/1 -> Multiport Switch/8
  1-D Lookup Table/1 -> Multiport Switch/5
  LowWarning/1 -> 1-D Lookup Table2/1
  HighWarning/1 -> 1-D Lookup Table3/1
  LowError/1 -> 1-D Lookup Table/1
  HighError/1 -> 1-D Lookup Table1/1

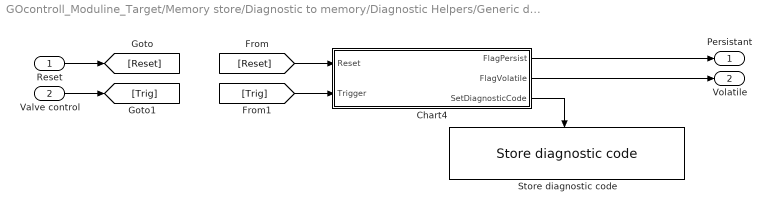
== system GOcontroll_Moduline_Target/Memory store/Diagnostic to memory/Diagnostic Helpers/Generic diagnostic ==
  Reset : Inport
  "Valve control " : Inport  Port=2
  Chart4 : Stateflow chart  TreatAsAtomicUnit=on
  Store diagnostic code : $bdroot/Memory store/Diagnostic to memory/Store diagnostic code  spn=spn  fmi=(0) Data valid but above normal operational range, most severe level (3)  TriggerType=rising
  Persistant : Outport
  Volatile : Outport  Port=2
  wires:
  Chart4/3(SetDiagnosticCode) -> Store diagnostic code/Trigger
  [Trig] -> Chart4/2(Trigger)
  Reset/1 -> [Reset]
  [Reset] -> Chart4/1(Reset)
  "Valve control "/1 -> [Trig]
  Chart4/1(FlagPersist) -> Persistant/1
  Chart4/2(FlagVolatile) -> Volatile/1
